simulink model "exp5"  (R2019b)
settings: Solver=VariableStepAuto  StartTime=0.0  StopTime=5/1000  RelTol=1e-3
libraries: dsparch4 x1, commsynccomp2 x1
settings Model: Creator=Lenovo  LastModifiedBy=Lenovo

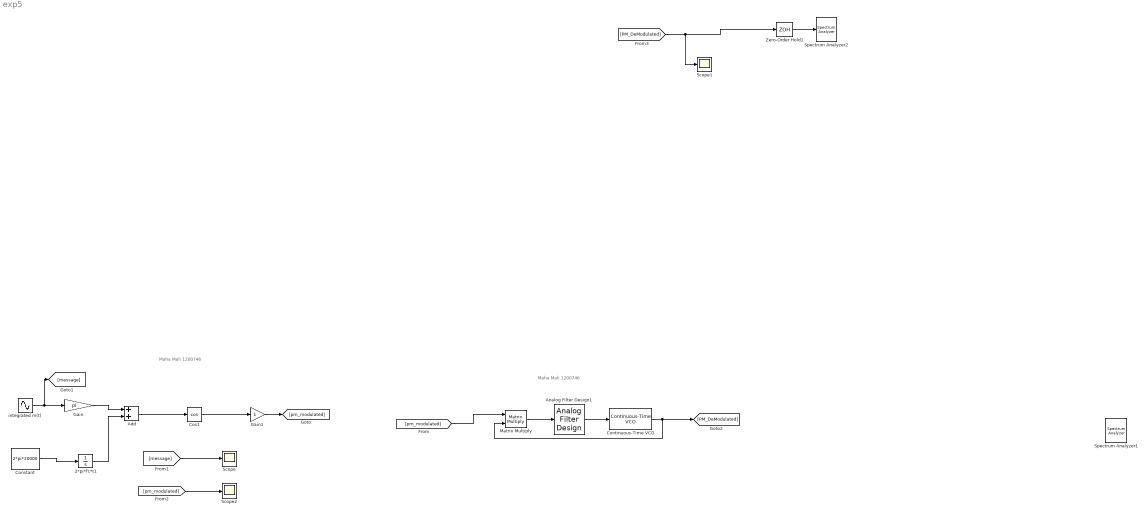
== system exp5 ==
  note: Maha Mali 1200746
  note: Maha Mali 1200746
  2*pi*fc*t1 : Integrator
  Add : Sum
  Analog Filter Design1 : dsparch4/Analog Filter Design  method=Butterworth  filttype=Lowpass  N=8  Wlo=pi*2*1000  Whi=80  Rp=2  Rs=40
  Constant : Constant  Value=2*pi*20000
  Continuous-Time VCO : commsynccomp2/Continuous-Time VCO  Ac=1  Fc=400  Kc=1  Ph=0
      settings: SourceProductName=Communications Toolbox  SourceProductBaseCode=CM
  Cos1 : Trigonometry  Operator=cos
  Gain : Gain  Gain=pi
  Gain1 : Gain
  Matrix Multiply : Product  Multiplication=Matrix(*)
  Scope : Scope
  Scope1 : Scope
  Scope2 : Scope
  Spectrum Analyzer1 : SpectrumAnalyzer
  Spectrum Analyzer2 : SpectrumAnalyzer
  Zero-Order Hold1 : ZeroOrderHold  SampleTime=1/(10*5e2)
  integrated m(t) : Sin  Frequency=500*pi*2  SampleTime=0
  wires:
  Gain/1 -> Add/1
  Cos1/1 -> Gain1/1
  integrated m(t)/1 -> [message], Gain/1
  Constant/1 -> 2*pi*fc*t1/1
  2*pi*fc*t1/1 -> Add/2
  Add/1 -> Cos1/1
  Gain1/1 -> [pm_modulated]
  [message] -> Scope/1
  [pm_modulated] -> Scope2/1
  Continuous-Time VCO/1 -> [PM_DeModulated], Matrix Multiply/2
  Matrix Multiply/1 -> Analog Filter Design1/1
  Analog Filter Design1/1 -> Continuous-Time VCO/1
  [pm_modulated] -> Matrix Multiply/1
  Zero-Order Hold1/1 -> Spectrum Analyzer2/1
  [PM_DeModulated] -> Scope1/1, Zero-Order Hold1/1
